simulink model "model_mondeo_offline1"  (Simulink 4.00)
settings: Solver=ode4  StartTime=t_0  StopTime=t_end  FixedStep=T_s  RelTol=1e-3
undefined symbols (not defined in the file or in its folder): nedc
libraries: lib_driveline_components x10, lib_VES_components x1
settings Model: LastModifiedBy=meifert  BlockReductionOpt=off

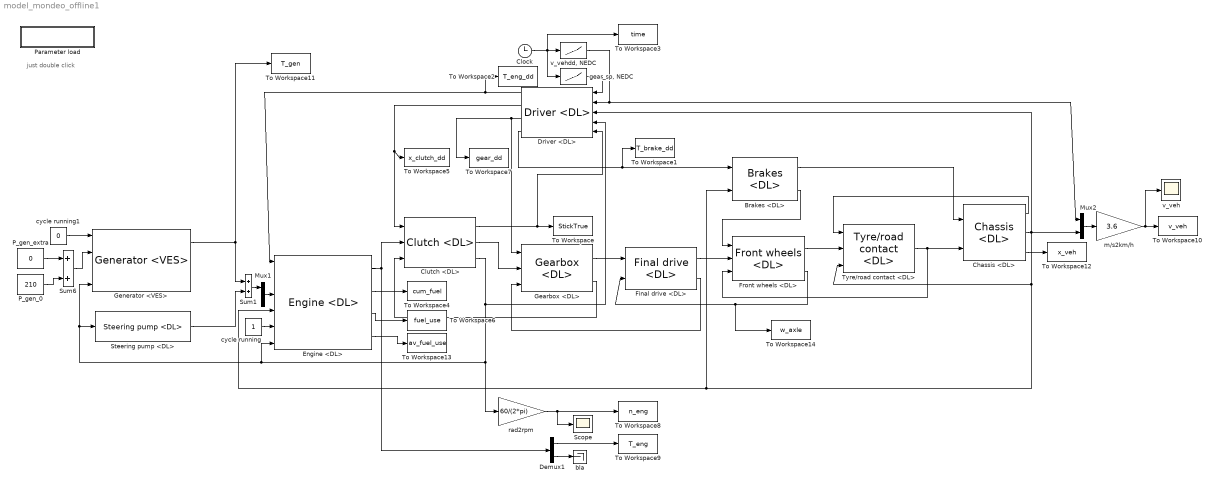
== system model_mondeo_offline1 ==
  note: just double click
  Brakes <DL> : lib_driveline_components/Brakes <DL>  AncestorBlock=|
      | lib_wheel/wheel and
      | axle <wh>/front/rear brake controller interface
      | (achievable)
      settings: RTWFcnNameOpts=Auto  RTWFileNameOpts=Auto
  Chassis <DL> : lib_driveline_components/Chassis <DL>
      settings: RTWFcnNameOpts=Auto  RTWFileNameOpts=Auto
  Clock : Clock
      settings: DisplayTime=off  Decimation=10
  Clutch <DL> : lib_driveline_components/Clutch <DL>
      settings: RTWFcnNameOpts=Auto  RTWFileNameOpts=Auto
  Demux1 : Demux  Outputs=2  BusSelectionMode=off
  Driver <DL> : lib_driveline_components/Driver <DL>  Orientation=left
      settings: RTWFcnNameOpts=Auto  RTWFileNameOpts=Auto
  Engine <DL> : lib_driveline_components/Engine <DL>
      settings: RTWFcnNameOpts=Auto  RTWFileNameOpts=Auto
  Final drive <DL> : lib_driveline_components/Final drive <DL>
      settings: RTWFcnNameOpts=Auto  RTWFileNameOpts=Auto
  Front wheels <DL> : lib_driveline_components/Front wheels <DL>
      settings: RTWFcnNameOpts=Auto  RTWFileNameOpts=Auto
  Gearbox <DL> : lib_driveline_components/Gearbox <DL>
      settings: RTWFcnNameOpts=Auto  RTWFileNameOpts=Auto
  Generator <VES> : lib_VES_components/Generator <VES>
      settings: RTWFcnNameOpts=Auto  RTWFileNameOpts=Auto
  Mux1 : Mux  Inputs=2
  Mux2 : Mux  Inputs=2
  P_gen_0 : Constant  Value=210
  P_gen_extra : Constant  Value=0
  Parameter load : Subsystem
      settings: OpenFcn=load_parms_offline  RTWFcnNameOpts=Auto  RTWFileNameOpts=Auto
      mask Display: disp('Load Parameters')
  Scope : Scope
      settings: TimeRange=50  YMin=500  YMax=2750  SaveToWorkspace=off  MaxDataPoints=5000
  Steering pump <DL> : lib_driveline_components/Steering pump <DL>
      settings: RTWFcnNameOpts=Auto  RTWFileNameOpts=Auto
  Sum1 : Sum  Inputs=++  SaturateOnIntegerOverflow=on
  Sum6 : Sum  Inputs=++  SaturateOnIntegerOverflow=on
  To Workspace : ToWorkspace  VariableName=StickTrue  SampleTime=-1  SaveFormat=Array
  To Workspace1 : ToWorkspace  VariableName=T_brake_dd  SampleTime=-1  SaveFormat=Array
  To Workspace10 : ToWorkspace  VariableName=v_veh  SampleTime=-1  SaveFormat=Array
  To Workspace11 : ToWorkspace  VariableName=T_gen  SampleTime=-1  SaveFormat=Array
  To Workspace12 : ToWorkspace  VariableName=x_veh  SampleTime=-1  SaveFormat=Array
  To Workspace13 : ToWorkspace  VariableName=av_fuel_use  SampleTime=-1  SaveFormat=Array
  To Workspace14 : ToWorkspace  VariableName=w_axle  SampleTime=-1  SaveFormat=Array
  To Workspace2 : ToWorkspace  VariableName=T_eng_dd  SampleTime=-1  SaveFormat=Array
  To Workspace3 : ToWorkspace  VariableName=time  SampleTime=-1  SaveFormat=Array
  To Workspace4 : ToWorkspace  VariableName=cum_fuel  SampleTime=-1  SaveFormat=Array
  To Workspace5 : ToWorkspace  VariableName=x_clutch_dd  SampleTime=-1  SaveFormat=Array
  To Workspace6 : ToWorkspace  VariableName=fuel_use  SampleTime=-1  SaveFormat=Array
  To Workspace7 : ToWorkspace  VariableName=gear_dd  SampleTime=-1  SaveFormat=Array
  To Workspace8 : ToWorkspace  VariableName=n_eng  SampleTime=-1  SaveFormat=Array
  To Workspace9 : ToWorkspace  VariableName=T_eng  SampleTime=-1  SaveFormat=Array
  Tyre/road contact <DL> : lib_driveline_components/Tyre//road contact <DL>
      settings: RTWFcnNameOpts=Auto  RTWFileNameOpts=Auto
  bla : Terminator
  cycle running : Constant  Value=1
  cycle running1 : Constant  Value=0
  "gear_sp, NEDC" : Lookup  InputValues=nedc.gearshift_points(:,1)  OutputValues=nedc.gearshift_points(:,2)
  m/s2km/h : Gain  Gain=3.6  Multiplication=Element-wise(K.*u)  SaturateOnIntegerOverflow=on
  rad2rpm : Gain  Gain=60/(2*pi)  Multiplication=Element-wise(K.*u)  SaturateOnIntegerOverflow=on
  v_veh : Scope
      settings: TimeRange=100  YMin=-2.5  YMax=35  SaveToWorkspace=off  SaveName=ScopeData  MaxDataPoints=5000
  "v_vehdd, NEDC" : Lookup  InputValues=nedc.speed(:,1)  OutputValues=nedc.speed(:,2)
  wires:
  Gearbox <DL>/1 -> Final drive <DL>/1
  Final drive <DL>/2 -> Gearbox <DL>/3
  Clutch <DL>/2 -> Gearbox <DL>/2
  Chassis <DL>/2 -> Driver <DL>/3, Brakes <DL>/2, Engine <DL>/4, Tyre/road contact <DL>/3, Mux2/2
  Front wheels <DL>/2 -> Final drive <DL>/2, To Workspace14/1
  rad2rpm/1 -> To Workspace8/1, Scope/1
  Demux1/1 -> To Workspace9/1
  Demux1/2 -> bla/1
  Clock/1 -> To Workspace3/1, "v_vehdd, NEDC"/1, "gear_sp, NEDC"/1
  Mux2/1 -> m/s2km/h/1
  "v_vehdd, NEDC"/1 -> Mux2/1, Driver <DL>/2
  Driver <DL>/4 -> To Workspace1/1, Brakes <DL>/1
  Driver <DL>/1 -> To Workspace2/1, Engine <DL>/1
  Driver <DL>/2 -> To Workspace5/1, Clutch <DL>/1
  Driver <DL>/3 -> Gearbox <DL>/1, To Workspace7/1
  m/s2km/h/1 -> To Workspace10/1, v_veh/1
  Brakes <DL>/1 -> Chassis <DL>/1
  Tyre/road contact <DL>/1 -> Front wheels <DL>/3, Chassis <DL>/2
  Front wheels <DL>/1 -> Tyre/road contact <DL>/2
  Chassis <DL>/1 -> Tyre/road contact <DL>/1
  Gearbox <DL>/2 -> Clutch <DL>/3
  Clutch <DL>/3 -> Driver <DL>/4, rad2rpm/1, Engine <DL>/6, Generator <VES>/4, Steering pump <DL>/1
  Clutch <DL>/1 -> To Workspace/1, Driver <DL>/5
  Brakes <DL>/2 -> Front wheels <DL>/1
  Final drive <DL>/1 -> Front wheels <DL>/2
  "gear_sp, NEDC"/1 -> Driver <DL>/1
  Mux1/1 -> Engine <DL>/3
  Engine <DL>/1 -> Clutch <DL>/2, Demux1/1
  P_gen_extra/1 -> Sum6/1
  Engine <DL>/3 -> To Workspace6/1
  cycle running/1 -> Engine <DL>/5
  Engine <DL>/2 -> To Workspace4/1
  Chassis <DL>/3 -> To Workspace12/1
  Engine <DL>/4 -> To Workspace13/1
  P_gen_0/1 -> Sum6/2
  Sum1/1 -> Mux1/1
  Steering pump <DL>/1 -> Sum1/2
  cycle running1/1 -> Generator <VES>/1
  Sum6/1 -> Generator <VES>/2
  Generator <VES>/1 -> Sum1/1, To Workspace11/1

== system model_mondeo_offline1/Parameter load ==
